simulink model "feedback"  (Simulink 7.7)
settings: Solver=ode4  StartTime=0.0  StopTime=1  FixedStep=0.001  RelTol=1e-3
settings Model: Creator=kononencheg  LastModifiedBy=kononencheg

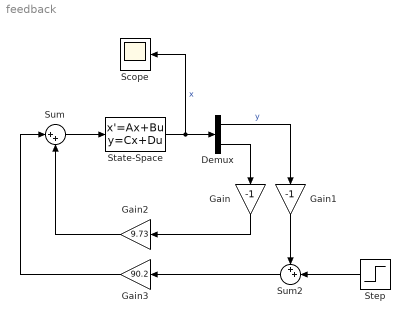
== system feedback ==
  Demux : Demux  Outputs=2
  Gain : Gain  Gain=-1
  Gain1 : Gain  Gain=-1
  Gain2 : Gain  Gain=9.73
  Gain3 : Gain  Gain=90.2
  Scope : Scope
      settings: TickLabels=on  SaveName=x
  State-Space : StateSpace  A=[0 1; -15 -5]  B=[0; 1]  C=[1, 0; 0, 1]  D=[0; 0]
  Step : Step  Time=0  SampleTime=0
  Sum : Sum  Inputs=|++
  Sum2 : Sum  Inputs=++|
  wires:
  Sum/1 -> State-Space/1
  State-Space/1 -> Demux/1, Scope/1  "x"
  Demux/2 -> Gain/1
  Demux/1 -> Gain1/1  "y"
  Gain1/1 -> Sum2/1
  Step/1 -> Sum2/2
  Gain/1 -> Gain2/1
  Sum2/1 -> Gain3/1
  Gain2/1 -> Sum/2
  Gain3/1 -> Sum/1
